simulink model "AUAV_V3_TestSensors"  (Simulink 8.5)
settings: Solver=FixedStepDiscrete  StartTime=0.0  StopTime=10.0  FixedStep=T  RelTol=1e-3
PreLoadFcn:
  | %T = 0.0025;
  | MavlinkBus;
  | mcuInit;
  | % Baro Altitude Computation
  | % =========================
  | basePressure = 98192.64;
  | baseTemp = 288.215;
  | lapseRate = -0.00198122;
  | baseHeight = 0;
undefined symbols (not defined in the file): A0, A14, A15, A2, A3, A4, A5, A6, accBiasRateLimit, apSampleTime, B0, bankCommandLimit, barAdjust, baroCutoff, baroCutTemp, baroOffset, baroScale, barTGain1, barTGain2, barTMean1, barTMean2, bda, bde, bdr, bdt, bICda, bICde, bICdr, bICdt, cubeAccelGain16405, cubeGyroGain16405, cubeMagGain16405, D0, D11, D7, D8, daLimit, data, daTrimMax, daTrimMin, deLimit, derivativesConstant, deTrimMax, deTrimMin, drLimit, drTrimMax, drTrimMin, dtLimit, dtTrimMax, dtTrimMin, F2, F3, G0, G13, G15, gaind, GS_location, gyroBiasRateLimit, IC1max, IPStar ... (+71)
libraries: MCHP_Blockset x152, simulink x84, SLUGS_Library x31, aerolibconvert2 x6, aerolibutil x4, aerolibtransform2 x3, dspmtrx3 x2, aerolibobsolete x2
(part 19 of 20)

== system AUAV_V3_TestSensors/Inner Loop/ Navigation/Navigation Encaps [updated 4.28.16]/Navigation/Normal WP  Navigation/Get Frenet/get WP Coord from Index2 ==
  WP Idx : Inport
  GS LLA : Inport  Port=2
  GS R_in : Inport  Port=3
  Demux1 : Demux  Outputs=3
  Environment Controller1 : simulink/Signal Routing/Environment Controller
  Geod2LTP2 : SLUGS_Library/Navigation/Geod2LTP
  Get WP Coord navsupport.c [updated 5.1.16] : MCHP_Blockset/User Functions/C Function Call  ParseFilesChkbx=off  ListFunctions1=Custom Function  Function1=void getWP(unsigned char idx, float* WPpos)  AddHeaderDeclaration=on  Function1Type=when block is updated (default)  Fct1BlockIn=idx  FctReturnBlockOut=on  Fct1BlockOut=WPpos[3]  DataCollected=0  ORDERING=None  SampleTime=-1  MCHP_MASTERLINK=|  PinDigitalInput=[]  PinDigitalOutput=[]  PinAnalogInput=[]
      | AUAV_V3_TestSensors/Microchip Master
      | AUAV V3 Board
      | Busy Flag on D2 (RA6)
  Get WP from idx SIM : Subsystem
  WP Coord : Outport
  wires:
  Geod2LTP2/1 -> Environment Controller1/2
  Get WP Coord navsupport.c [updated 5.1.16]/1 -> Demux1/1
  Demux1/3 -> Geod2LTP2/5
  Demux1/2 -> Geod2LTP2/4
  Demux1/1 -> Geod2LTP2/3
  Get WP from idx SIM/1(Out1) -> Environment Controller1/1
  Environment Controller1/1 -> WP Coord/1
  GS R_in/1 -> Get WP from idx SIM/2(GS ECEF), Geod2LTP2/2
  GS LLA/1 -> Get WP from idx SIM/1(GS LLA), Geod2LTP2/1
  WP Idx/1 -> Get WP from idx SIM/3(idx), Get WP Coord navsupport.c [updated 5.1.16]/1

== system AUAV_V3_TestSensors/Inner Loop/ Navigation/Navigation Encaps [updated 4.28.16]/Navigation/Normal WP  Navigation/On WP Enable/Subsystem ==
  GS LLA : Inport
  GS R_in : Inport  Port=2
  Compute Frenet : Subsystem  AncestorBlock=SLUGS_Library/Navigation/Compute Frenet
  Constant : Constant  OutDataTypeStr=uint8  SampleTime=0.01
  Constant1 : Constant  Value=2  OutDataTypeStr=uint8  SampleTime=0.01
  GS LLA_1 : InportShadow
  GS R_in_1 : InportShadow  Port=2
  Terminator : Terminator
  get WP Coord from Index : Subsystem  AncestorBlock=SLUGS_Library/Navigation/get WP Coord from Index
  get WP Coord from Index1 : Subsystem  AncestorBlock=SLUGS_Library/Navigation/get WP Coord from Index
  WP0 : Outport
  T1 : Outport  Port=2
  wires:
  Constant/1 -> get WP Coord from Index/1(WP Idx)
  Compute Frenet/2(N) -> Terminator/1
  Compute Frenet/1(T) -> T1/1
  GS LLA/1 -> get WP Coord from Index/2(GS LLA)
  GS R_in/1 -> get WP Coord from Index/3(GS R_in)
  get WP Coord from Index/1(WP Coord) -> WP0/1, Compute Frenet/1(Pos 1)
  get WP Coord from Index1/1(WP Coord) -> Compute Frenet/2(Pos 2)
  Constant1/1 -> get WP Coord from Index1/1(WP Idx)
  GS LLA_1/1 -> get WP Coord from Index1/2(GS LLA)
  GS R_in_1/1 -> get WP Coord from Index1/3(GS R_in)

== system AUAV_V3_TestSensors/Inner Loop/ Navigation/Navigation Encaps [updated 4.28.16]/Navigation/Normal WP  Navigation/Vector Norm/dsPIC_SQRT ==
  x : Inport
  Environment Controller : simulink/Signal Routing/Environment Controller
  Math Function1 : Math  Operator=sqrt  SaturateOnIntegerOverflow=on
  mySqrt() apUtils.c [updated 5.1.16] : MCHP_Blockset/User Functions/C Function Call  ParseFilesChkbx=off  ListFunctions1=Custom Function  Function1=float mySqrt(float x)  AddHeaderDeclaration=on  Function1Type=when block is updated (default)  Fct1BlockIn=x  FctReturnBlockOut=on  DataCollected=0  ORDERING=None  SampleTime=-1  MCHP_MASTERLINK=|  PinDigitalInput=[]  PinDigitalOutput=[]  PinAnalogInput=[]
      | AUAV_V3_TestSensors/Microchip Master
      | AUAV V3 Board
      | Busy Flag on D2 (RA6)
  negprotect : MATLAB Function  TreatAsAtomicUnit=on
  sqrt(x) : Outport
  wires:
  x/1 -> negprotect/1(val)
  negprotect/1(zpVal) -> Math Function1/1, mySqrt() apUtils.c [updated 5.1.16]/1
  Environment Controller/1 -> sqrt(x)/1
  Math Function1/1 -> Environment Controller/1
  mySqrt() apUtils.c [updated 5.1.16]/1 -> Environment Controller/2

== system AUAV_V3_TestSensors/Inner Loop/ Navigation/Navigation Encaps [updated 4.28.16]/Navigation/RTB/Follow Mobile Navigation/Vector Norm/dsPIC_SQRT ==
  x : Inport
  Environment Controller : simulink/Signal Routing/Environment Controller
  Math Function1 : Math  Operator=sqrt  SaturateOnIntegerOverflow=on
  mySqrt() apUtils.c [updated 5.1.16] : MCHP_Blockset/User Functions/C Function Call  ParseFilesChkbx=off  ListFunctions1=Custom Function  Function1=float mySqrt(float x)  AddHeaderDeclaration=on  Function1Type=when block is updated (default)  Fct1BlockIn=x  FctReturnBlockOut=on  DataCollected=0  ORDERING=None  SampleTime=-1  MCHP_MASTERLINK=|  PinDigitalInput=[]  PinDigitalOutput=[]  PinAnalogInput=[]
      | AUAV_V3_TestSensors/Microchip Master
      | AUAV V3 Board
      | Busy Flag on D2 (RA6)
  negprotect : MATLAB Function  TreatAsAtomicUnit=on
  sqrt(x) : Outport
  wires:
  x/1 -> negprotect/1(val)
  negprotect/1(zpVal) -> Math Function1/1, mySqrt() apUtils.c [updated 5.1.16]/1
  Environment Controller/1 -> sqrt(x)/1
  Math Function1/1 -> Environment Controller/1
  mySqrt() apUtils.c [updated 5.1.16]/1 -> Environment Controller/2

== system AUAV_V3_TestSensors/Inner Loop/ Navigation/Navigation Encaps [updated 4.28.16]/Navigation/Recent Enable/Grab Upon Enable/Compute GS Location ==
  GS Location : Inport
  Demux : Demux  Outputs=3
  Geod2ECEF1 : Subsystem  mask{Re=6378137, Rp=6356752.3142}
      mask prompts: Re "Enter equatorial radius, m"; Rp "Enter polar radius,m"
  Mux1 : Mux  Inputs=2
  Mux2 : Mux  Inputs=3
  "Lon, Lat" : Outport
  R_in : Outport  Port=2
  wires:
  Mux2/1 -> R_in/1  "R_in"
  Mux1/1 -> "Lon, Lat"/1
  GS Location/1 -> Demux/1
  Demux/3 -> Mux1/1, Geod2ECEF1/3(lon,deg)
  Demux/2 -> Mux1/2, Geod2ECEF1/2("lat, deg")
  Demux/1 -> Geod2ECEF1/1("height, m")
  Geod2ECEF1/2("Ye, m ") -> Mux2/2
  Geod2ECEF1/1("Xe, m ") -> Mux2/1
  Geod2ECEF1/3("Ze, m ") -> Mux2/3

== system AUAV_V3_TestSensors/Inner Loop/ Navigation/Navigation Encaps [updated 4.28.16]/Navigation/Recent Enable/Subsystem/Detect Rising Edge ==
  In1 : Inport
  Delay : Delay  DelayLength=1
  Logical Operator : Logic  AllPortsSameDT=off  OutDataTypeStr=boolean
  Relational Operator : RelationalOperator  Operator=~=  OutDataTypeStr=boolean
  Out1 : Outport
  wires:
  Delay/1 -> Relational Operator/1
  Relational Operator/1 -> Logical Operator/1
  In1/1 -> Delay/1, Relational Operator/2, Logical Operator/2
  Logical Operator/1 -> Out1/1

== system AUAV_V3_TestSensors/Position_and_Attitude_Filter/Position Filter/BlendPosVel/CompFiltRate/1D Filter1/Filter2 ==
  In1 : Inport
  Discrete Zero-Pole : DiscreteZeroPole  Zeros=zerosd  Poles=polesd  Gain=gaind  SampleTime=SampleTime
  Out1 : Outport
  wires:
  Discrete Zero-Pole/1 -> Out1/1
  In1/1 -> Discrete Zero-Pole/1

== system AUAV_V3_TestSensors/Position_and_Attitude_Filter/Position Filter/BlendPosVel/CompFiltRate1/1D Filter1/Filter2 ==
  In1 : Inport
  Discrete Zero-Pole : DiscreteZeroPole  Zeros=zerosd  Poles=polesd  Gain=gaind  SampleTime=SampleTime
  Out1 : Outport
  wires:
  Discrete Zero-Pole/1 -> Out1/1
  In1/1 -> Discrete Zero-Pole/1

== system AUAV_V3_TestSensors/Position_and_Attitude_Filter/Position Filter/BlendPosVel/CompRateOnly/1D Filter1/Filter2 ==
  In1 : Inport
  Discrete Zero-Pole : DiscreteZeroPole  Zeros=zerosd  Poles=polesd  Gain=gaind  SampleTime=SampleTime
  Out1 : Outport
  wires:
  Discrete Zero-Pole/1 -> Out1/1
  In1/1 -> Discrete Zero-Pole/1

== system AUAV_V3_TestSensors/Sensor_Data_Adapter/Sensor Suite/Low Pass Filtering,Temperature Compensation and Calibration/Baro Altimeter/Initial Baro Bias/Low Pass8 ==
  In1 : Inport
  Discrete Zero-Pole : DiscreteZeroPole  Zeros=zerosd  Poles=polesd  Gain=gaind  SampleTime=SampleTime
  Out1 : Outport
  wires:
  In1/1 -> Discrete Zero-Pole/1
  Discrete Zero-Pole/1 -> Out1/1

== system AUAV_V3_TestSensors/Inner Loop/ Navigation/Navigation Encaps [updated 4.28.16]/Navigation/Circle Navigation/Intersection. Circular Navigation/Compute Angle Between Vectors1/Vector Norm ==
  Vector : Inport
  dsPIC Dot Product : SLUGS_Library/dsPIC Dot Product
  dsPIC_SQRT : Subsystem  AncestorBlock=SLUGS_Library/dsPIC_SQRT
  Norm : Outport
  wires:
  dsPIC_SQRT/1(sqrt(x)) -> Norm/1
  Vector/1 -> dsPIC Dot Product/2, dsPIC Dot Product/1
  dsPIC Dot Product/1 -> dsPIC_SQRT/1(x)

== system AUAV_V3_TestSensors/Inner Loop/ Navigation/Navigation Encaps [updated 4.28.16]/Navigation/Circle Navigation/Intersection. Circular Navigation/Compute Angle Between Vectors1/dsPIC_acos ==
  x : Inport
  Environment Controller : simulink/Signal Routing/Environment Controller
  Trigonometric Function : Trigonometry  Operator=acos
  myAcos() apUtils.c [updated 5.1.16] : MCHP_Blockset/User Functions/C Function Call  ParseFilesChkbx=off  ListFunctions1=Custom Function  Function1=float myAcos(float x)  AddHeaderDeclaration=off  Function1Type=when block is updated (default)  Fct1BlockIn=x  FctReturnBlockOut=on  DataCollected=0  ORDERING=None  SampleTime=-1  MCHP_MASTERLINK=|  PinDigitalInput=[]  PinDigitalOutput=[]  PinAnalogInput=[]
      | AUAV_V3_TestSensors/Microchip Master
      | AUAV V3 Board
      | Busy Flag on D2 (RA6)
  acos(x) : Outport
  wires:
  Environment Controller/1 -> acos(x)/1
  myAcos() apUtils.c [updated 5.1.16]/1 -> Environment Controller/2
  Trigonometric Function/1 -> Environment Controller/1
  x/1 -> Trigonometric Function/1, myAcos() apUtils.c [updated 5.1.16]/1

== system AUAV_V3_TestSensors/Inner Loop/ Navigation/Navigation Encaps [updated 4.28.16]/Navigation/Circle Navigation/Intersection. Circular Navigation/Compute Angle Between Vectors2/Vector Norm ==
  Vector : Inport
  dsPIC Dot Product : SLUGS_Library/dsPIC Dot Product
  dsPIC_SQRT : Subsystem  AncestorBlock=SLUGS_Library/dsPIC_SQRT
  Norm : Outport
  wires:
  dsPIC_SQRT/1(sqrt(x)) -> Norm/1
  Vector/1 -> dsPIC Dot Product/2, dsPIC Dot Product/1
  dsPIC Dot Product/1 -> dsPIC_SQRT/1(x)

== system AUAV_V3_TestSensors/Inner Loop/ Navigation/Navigation Encaps [updated 4.28.16]/Navigation/Circle Navigation/Intersection. Circular Navigation/Compute Angle Between Vectors2/dsPIC_acos ==
  x : Inport
  Environment Controller : simulink/Signal Routing/Environment Controller
  Trigonometric Function : Trigonometry  Operator=acos
  myACos() apUtils.c [updated 5.1.16] : MCHP_Blockset/User Functions/C Function Call  ParseFilesChkbx=off  ListFunctions1=Custom Function  Function1=float myAcos(float x)  AddHeaderDeclaration=off  Function1Type=when block is updated (default)  Fct1BlockIn=x  FctReturnBlockOut=on  DataCollected=0  ORDERING=None  SampleTime=-1  MCHP_MASTERLINK=|  PinDigitalInput=[]  PinDigitalOutput=[]  PinAnalogInput=[]
      | AUAV_V3_TestSensors/Microchip Master
      | AUAV V3 Board
      | Busy Flag on D2 (RA6)
  acos(x) : Outport
  wires:
  Environment Controller/1 -> acos(x)/1
  myACos() apUtils.c [updated 5.1.16]/1 -> Environment Controller/2
  Trigonometric Function/1 -> Environment Controller/1
  x/1 -> Trigonometric Function/1, myACos() apUtils.c [updated 5.1.16]/1

== system AUAV_V3_TestSensors/Inner Loop/ Navigation/Navigation Encaps [updated 4.28.16]/Navigation/L2+/Get Sin, Cos eta/Get  Groundspeed/Vector Norm ==
  Vector : Inport
  dsPIC Dot Product : SLUGS_Library/dsPIC Dot Product
  dsPIC_SQRT : Subsystem  AncestorBlock=SLUGS_Library/dsPIC_SQRT
  Norm : Outport
  wires:
  dsPIC_SQRT/1(sqrt(x)) -> Norm/1
  Vector/1 -> dsPIC Dot Product/2, dsPIC Dot Product/1
  dsPIC Dot Product/1 -> dsPIC_SQRT/1(x)

== system AUAV_V3_TestSensors/Inner Loop/ Navigation/Navigation Encaps [updated 4.28.16]/Navigation/Normal WP  Navigation/Compute WP Switching Trigger/Compute  Projection/Protect NaNs ==
  In1 : Inport
  Integer Delay3 : Delay  DelayLength=1  InputProcessing=Inherited  SampleTime=T
  Relational Operator2 : RelationalOperator  Operator===  OutDataTypeStr=uint(8)
  Switch3 : Switch  Criteria=u2 > Threshold  Threshold=0.3  SampleTime=.01
  Out1 : Outport
  wires:
  Relational Operator2/1 -> Switch3/2
  In1/1 -> Switch3/1, Relational Operator2/1, Relational Operator2/2
  Switch3/1 -> Integer Delay3/1, Out1/1
  Integer Delay3/1 -> Switch3/3

== system AUAV_V3_TestSensors/Inner Loop/ Navigation/Navigation Encaps [updated 4.28.16]/Navigation/Normal WP  Navigation/Get Frenet/Compute Frenet/Normalize Vector ==
  Vector : Inport
  Divide : Product  Inputs=*/
  Vector Norm : Subsystem  AncestorBlock=SLUGS_Library/Vector Norm
  Zero Bound : Saturate  UpperLimit=inf  LowerLimit=0.001
  Normalized : Outport
  wires:
  Vector/1 -> Vector Norm/1(Vector), Divide/1
  Vector Norm/1(Norm) -> Zero Bound/1
  Zero Bound/1 -> Divide/2
  Divide/1 -> Normalized/1

== system AUAV_V3_TestSensors/Inner Loop/ Navigation/Navigation Encaps [updated 4.28.16]/Navigation/Normal WP  Navigation/Get Frenet/Compute Frenet/Normalize Vector  ==
  Vector : Inport
  Divide : Product  Inputs=*/
  Vector Norm : Subsystem  AncestorBlock=SLUGS_Library/Vector Norm
  Zero Bound : Saturate  UpperLimit=inf  LowerLimit=0.001
  Normalized : Outport
  wires:
  Vector/1 -> Vector Norm/1(Vector), Divide/1
  Vector Norm/1(Norm) -> Zero Bound/1
  Zero Bound/1 -> Divide/2
  Divide/1 -> Normalized/1

== system AUAV_V3_TestSensors/Inner Loop/ Navigation/Navigation Encaps [updated 4.28.16]/Navigation/Normal WP  Navigation/Get Frenet/get WP Coord from Index1/Get WP from idx SIM ==
  GS LLA : Inport
  GS ECEF : Inport  Port=2
  idx : Inport  Port=3
  Constant : Constant  Value=latlong_WP  OutDataTypeStr=uint8  SampleTime=0.01
  Constant1 : Constant  Value=Ypoints  OutDataTypeStr=double  SampleTime=0.01
  Constant2 : Constant  Value=Xpoints  OutDataTypeStr=double  SampleTime=0.01
  Constant3 : Constant  Value=Zpoints  OutDataTypeStr=double  SampleTime=0.01
  Data Type Conversion : DataTypeConversion  OutDataTypeStr=double
  Data Type Conversion1 : DataTypeConversion  OutDataTypeStr=single
  Demux : Demux  Outputs=3
  Geod2LTP1 : SLUGS_Library/Navigation/Geod2LTP
  Mux : Mux  Inputs=3
  Switch : Switch  Criteria=u2 > Threshold  Threshold=0.3  ZeroCross=off
  Zero out Z1 : MATLAB Function  TreatAsAtomicUnit=on
  Zero out Z2 : MATLAB Function  TreatAsAtomicUnit=on
  Zero out Z3 : MATLAB Function  TreatAsAtomicUnit=on
  Out1 : Outport
  wires:
  Constant2/1 -> Zero out Z2/2(vect)
  Constant3/1 -> Zero out Z3/2(vect)
  Constant1/1 -> Zero out Z1/2(vect)
  Switch/1 -> Out1/1
  idx/1 -> Data Type Conversion/1
  GS ECEF/1 -> Geod2LTP1/2
  GS LLA/1 -> Geod2LTP1/1
  Data Type Conversion1/1 -> Demux/1, Switch/3
  Geod2LTP1/1 -> Switch/1
  Demux/3 -> Geod2LTP1/5
  Demux/2 -> Geod2LTP1/4
  Demux/1 -> Geod2LTP1/3
  Constant/1 -> Switch/2
  Mux/1 -> Data Type Conversion1/1
  Zero out Z3/1(y) -> Mux/3
  Zero out Z1/1(y) -> Mux/2
  Zero out Z2/1(y) -> Mux/1
  Data Type Conversion/1 -> Zero out Z3/1(idx), Zero out Z1/1(idx), Zero out Z2/1(idx)

== system AUAV_V3_TestSensors/Inner Loop/ Navigation/Navigation Encaps [updated 4.28.16]/Navigation/Normal WP  Navigation/Get Frenet/get WP Coord from Index2/Get WP from idx SIM ==
  GS LLA : Inport
  GS ECEF : Inport  Port=2
  idx : Inport  Port=3
  Constant : Constant  Value=latlong_WP  OutDataTypeStr=uint8  SampleTime=0.01
  Constant1 : Constant  Value=Ypoints  OutDataTypeStr=double  SampleTime=0.01
  Constant2 : Constant  Value=Xpoints  OutDataTypeStr=double  SampleTime=0.01
  Constant3 : Constant  Value=Zpoints  OutDataTypeStr=double  SampleTime=0.01
  Data Type Conversion : DataTypeConversion  OutDataTypeStr=double
  Data Type Conversion1 : DataTypeConversion  OutDataTypeStr=single
  Demux : Demux  Outputs=3
  Geod2LTP1 : SLUGS_Library/Navigation/Geod2LTP
  Mux : Mux  Inputs=3
  Switch : Switch  Criteria=u2 > Threshold  Threshold=0.3  ZeroCross=off
  Zero out Z1 : MATLAB Function  TreatAsAtomicUnit=on
  Zero out Z2 : MATLAB Function  TreatAsAtomicUnit=on
  Zero out Z3 : MATLAB Function  TreatAsAtomicUnit=on
  Out1 : Outport
  wires:
  Constant2/1 -> Zero out Z2/2(vect)
  Constant3/1 -> Zero out Z3/2(vect)
  Constant1/1 -> Zero out Z1/2(vect)
  Switch/1 -> Out1/1
  idx/1 -> Data Type Conversion/1
  GS ECEF/1 -> Geod2LTP1/2
  GS LLA/1 -> Geod2LTP1/1
  Data Type Conversion1/1 -> Demux/1, Switch/3
  Geod2LTP1/1 -> Switch/1
  Demux/3 -> Geod2LTP1/5
  Demux/2 -> Geod2LTP1/4
  Demux/1 -> Geod2LTP1/3
  Constant/1 -> Switch/2
  Mux/1 -> Data Type Conversion1/1
  Zero out Z3/1(y) -> Mux/3
  Zero out Z1/1(y) -> Mux/2
  Zero out Z2/1(y) -> Mux/1
  Data Type Conversion/1 -> Zero out Z3/1(idx), Zero out Z1/1(idx), Zero out Z2/1(idx)

== system AUAV_V3_TestSensors/Inner Loop/ Navigation/Navigation Encaps [updated 4.28.16]/Navigation/Normal WP  Navigation/On WP Enable/Subsystem/Compute Frenet ==
  Pos 1 : Inport
  Pos 2 : Inport  Port=2
  Add : Sum  Inputs=-+
  Normalize Vector : Subsystem  AncestorBlock=SLUGS_Library/Navigation/Normalize Vector
  "Normalize Vector " : Subsystem  AncestorBlock=SLUGS_Library/Navigation/Normalize Vector
  Select N  Terms : MATLAB Function  TreatAsAtomicUnit=on
  T : Outport
  N : Outport  Port=2
  wires:
  "Normalize Vector "/1(Normalized) -> N/1
  Select N  Terms/1(N) -> "Normalize Vector "/1(Vector)
  Normalize Vector/1(Normalized) -> Select N  Terms/1(T), T/1
  Add/1 -> Normalize Vector/1(Vector)
  Pos 2/1 -> Add/2
  Pos 1/1 -> Add/1

== system AUAV_V3_TestSensors/Inner Loop/ Navigation/Navigation Encaps [updated 4.28.16]/Navigation/Normal WP  Navigation/On WP Enable/Subsystem/get WP Coord from Index ==
  WP Idx : Inport
  GS LLA : Inport  Port=2
  GS R_in : Inport  Port=3
  Demux1 : Demux  Outputs=3
  Environment Controller1 : simulink/Signal Routing/Environment Controller
  Geod2LTP2 : SLUGS_Library/Navigation/Geod2LTP
  Get WP Coord navsupport.c [updated 5.1.16] : MCHP_Blockset/User Functions/C Function Call  ParseFilesChkbx=off  ListFunctions1=Custom Function  Function1=void getWP(unsigned char idx, float* WPpos)  AddHeaderDeclaration=on  Function1Type=when block is updated (default)  Fct1BlockIn=idx  FctReturnBlockOut=on  Fct1BlockOut=WPpos[3]  DataCollected=0  ORDERING=None  SampleTime=-1  MCHP_MASTERLINK=|  PinDigitalInput=[]  PinDigitalOutput=[]  PinAnalogInput=[]
      | AUAV_V3_TestSensors/Microchip Master
      | AUAV V3 Board
      | Busy Flag on D2 (RA6)
  Get WP from idx SIM : Subsystem
  WP Coord : Outport
  wires:
  Geod2LTP2/1 -> Environment Controller1/2
  Get WP Coord navsupport.c [updated 5.1.16]/1 -> Demux1/1
  Demux1/3 -> Geod2LTP2/5
  Demux1/2 -> Geod2LTP2/4
  Demux1/1 -> Geod2LTP2/3
  Get WP from idx SIM/1(Out1) -> Environment Controller1/1
  Environment Controller1/1 -> WP Coord/1
  GS R_in/1 -> Get WP from idx SIM/2(GS ECEF), Geod2LTP2/2
  GS LLA/1 -> Get WP from idx SIM/1(GS LLA), Geod2LTP2/1
  WP Idx/1 -> Get WP from idx SIM/3(idx), Get WP Coord navsupport.c [updated 5.1.16]/1

== system AUAV_V3_TestSensors/Inner Loop/ Navigation/Navigation Encaps [updated 4.28.16]/Navigation/Normal WP  Navigation/On WP Enable/Subsystem/get WP Coord from Index1 ==
  WP Idx : Inport
  GS LLA : Inport  Port=2
  GS R_in : Inport  Port=3
  Demux1 : Demux  Outputs=3
  Environment Controller1 : simulink/Signal Routing/Environment Controller
  Geod2LTP2 : SLUGS_Library/Navigation/Geod2LTP
  Get WP Coord navsupport.c [updated 5.1.16] : MCHP_Blockset/User Functions/C Function Call  ParseFilesChkbx=off  ListFunctions1=Custom Function  Function1=void getWP(unsigned char idx, float* WPpos)  AddHeaderDeclaration=on  Function1Type=when block is updated (default)  Fct1BlockIn=idx  FctReturnBlockOut=on  Fct1BlockOut=WPpos[3]  DataCollected=0  ORDERING=None  SampleTime=-1  MCHP_MASTERLINK=|  PinDigitalInput=[]  PinDigitalOutput=[]  PinAnalogInput=[]
      | AUAV_V3_TestSensors/Microchip Master
      | AUAV V3 Board
      | Busy Flag on D2 (RA6)
  Get WP from idx SIM : Subsystem
  WP Coord : Outport
  wires:
  Geod2LTP2/1 -> Environment Controller1/2
  Get WP Coord navsupport.c [updated 5.1.16]/1 -> Demux1/1
  Demux1/3 -> Geod2LTP2/5
  Demux1/2 -> Geod2LTP2/4
  Demux1/1 -> Geod2LTP2/3
  Get WP from idx SIM/1(Out1) -> Environment Controller1/1
  Environment Controller1/1 -> WP Coord/1
  GS R_in/1 -> Get WP from idx SIM/2(GS ECEF), Geod2LTP2/2
  GS LLA/1 -> Get WP from idx SIM/1(GS LLA), Geod2LTP2/1
  WP Idx/1 -> Get WP from idx SIM/3(idx), Get WP Coord navsupport.c [updated 5.1.16]/1

== system AUAV_V3_TestSensors/Inner Loop/ Navigation/Navigation Encaps [updated 4.28.16]/Navigation/Recent Enable/Grab Upon Enable/Compute GS Location/Geod2ECEF1 ==
  "height, m" : Inport
  "lat, deg" : Inport  Port=2
  lon,deg : Inport  Port=3
  (Rh+h)cos(phi)*cos(lamb)=Xe : Product  Inputs=3  OutDataTypeStr=single  SaturateOnIntegerOverflow=on  InputSameDT=on
  (Rh+h)cos(phi)*sin(lamb)=Ye : Product  Inputs=3  OutDataTypeStr=single  SaturateOnIntegerOverflow=on  InputSameDT=on
  Deg2R : Gain  Gain=pi/180  OutDataTypeStr=float('single')  SaturateOnIntegerOverflow=on  ParamDataTypeStr=Inherit: Same as input
  Deg2R1 : Gain  Gain=pi/180  OutDataTypeStr=float('single')  SaturateOnIntegerOverflow=on  ParamDataTypeStr=Inherit: Same as input
  Product1 : Product  SaturateOnIntegerOverflow=on  InputSameDT=on  OutDataTypeStr=Inherit: Same as first input
  Re=equatorial radius : Constant  Value=Re  OutDataTypeStr=single
  Rh : Product  Inputs=*/  OutDataTypeStr=single  SaturateOnIntegerOverflow=on  InputSameDT=on
  Rh(1-e^2) : Product  OutDataTypeStr=single  SaturateOnIntegerOverflow=on  InputSameDT=on
  Sum1 : Sum  Inputs=+-|  SaturateOnIntegerOverflow=on  InputSameDT=on  OutDataTypeStr=Inherit: Same as first input
  Sum2 : Sum  SaturateOnIntegerOverflow=on  InputSameDT=on  OutDataTypeStr=Inherit: Same as first input
      settings: AttributesFormatString=Rh+h
  Sum3 : Sum  Inputs=|+-  SaturateOnIntegerOverflow=on  InputSameDT=on  OutDataTypeStr=Inherit: Same as first input
  Sum4 : Sum  OutDataTypeStr=single  SaturateOnIntegerOverflow=on  InputSameDT=on
      settings: AttributesFormatString=(1-e^2)Rh+h
  Ze : Product  OutDataTypeStr=single  SaturateOnIntegerOverflow=on  InputSameDT=on
  const : Constant  OutDataTypeStr=single
  const1 : Constant  OutDataTypeStr=single
  cos(lamb) : Trigonometry  Operator=cos
  cos(phi) : Trigonometry  Operator=cos
  eccentricity^2 : Subsystem
  f : Fcn  Expr=sqrt(u(1))
  sin(lamb) : Trigonometry
  sin(phi) : Trigonometry
  sin(phi)^2 : Product  SaturateOnIntegerOverflow=on  InputSameDT=on  OutDataTypeStr=Inherit: Same as first input
  "Xe, m " : Outport
  "Ye, m " : Outport  Port=2
  "Ze, m " : Outport  Port=3
  wires:
  "lat, deg"/1 -> Deg2R/1
  sin(phi)/1 -> sin(phi)^2/1, sin(phi)^2/2, Ze/1
  f/1 -> Rh/2
  Re=equatorial radius/1 -> Rh/1
  Rh/1 -> Sum2/2, Rh(1-e^2)/2
  Product1/1 -> Sum1/2
  Sum1/1 -> f/1
  const/1 -> Sum1/1
  "height, m"/1 -> Sum4/2, Sum2/1
  eccentricity^2/1(e^2) -> Product1/1, Sum3/2
  sin(phi)^2/1 -> Product1/2
  const1/1 -> Sum3/1
  Sum3/1 -> Rh(1-e^2)/1  "1-e^2"
  Rh(1-e^2)/1 -> Sum4/1
  Sum4/1 -> Ze/2
  lon,deg/1 -> Deg2R1/1
  cos(phi)/1 -> (Rh+h)cos(phi)*cos(lamb)=Xe/2, (Rh+h)cos(phi)*sin(lamb)=Ye/2
  cos(lamb)/1 -> (Rh+h)cos(phi)*cos(lamb)=Xe/3
  sin(lamb)/1 -> (Rh+h)cos(phi)*sin(lamb)=Ye/3
  Ze/1 -> "Ze, m "/1
  Deg2R/1 -> cos(phi)/1, sin(phi)/1
  Deg2R1/1 -> cos(lamb)/1, sin(lamb)/1
  Sum2/1 -> (Rh+h)cos(phi)*sin(lamb)=Ye/1, (Rh+h)cos(phi)*cos(lamb)=Xe/1
  (Rh+h)cos(phi)*cos(lamb)=Xe/1 -> "Xe, m "/1
  (Rh+h)cos(phi)*sin(lamb)=Ye/1 -> "Ye, m "/1

== system AUAV_V3_TestSensors/Inner Loop/ Navigation/Navigation Encaps [updated 4.28.16]/Navigation/Circle Navigation/Intersection. Circular Navigation/Compute Angle Between Vectors1/Vector Norm/dsPIC_SQRT ==
  x : Inport
  Environment Controller : simulink/Signal Routing/Environment Controller
  Math Function1 : Math  Operator=sqrt  SaturateOnIntegerOverflow=on
  mySqrt() apUtils.c [updated 5.1.16] : MCHP_Blockset/User Functions/C Function Call  ParseFilesChkbx=off  ListFunctions1=Custom Function  Function1=float mySqrt(float x)  AddHeaderDeclaration=off  Function1Type=when block is updated (default)  Fct1BlockIn=x  FctReturnBlockOut=on  DataCollected=0  ORDERING=None  SampleTime=-1  MCHP_MASTERLINK=|  PinDigitalInput=[]  PinDigitalOutput=[]  PinAnalogInput=[]
      | AUAV_V3_TestSensors/Microchip Master
      | AUAV V3 Board
      | Busy Flag on D2 (RA6)
  negprotect : MATLAB Function  TreatAsAtomicUnit=on
  sqrt(x) : Outport
  wires:
  x/1 -> negprotect/1(val)
  negprotect/1(zpVal) -> Math Function1/1, mySqrt() apUtils.c [updated 5.1.16]/1
  Environment Controller/1 -> sqrt(x)/1
  Math Function1/1 -> Environment Controller/1
  mySqrt() apUtils.c [updated 5.1.16]/1 -> Environment Controller/2

== system AUAV_V3_TestSensors/Inner Loop/ Navigation/Navigation Encaps [updated 4.28.16]/Navigation/Circle Navigation/Intersection. Circular Navigation/Compute Angle Between Vectors2/Vector Norm/dsPIC_SQRT ==
  x : Inport
  Environment Controller : simulink/Signal Routing/Environment Controller
  Math Function1 : Math  Operator=sqrt  SaturateOnIntegerOverflow=on
  mySqrt() apUtils.c [updated 5.1.16] : MCHP_Blockset/User Functions/C Function Call  ParseFilesChkbx=off  ListFunctions1=Custom Function  Function1=float mySqrt(float x)  AddHeaderDeclaration=off  Function1Type=when block is updated (default)  Fct1BlockIn=x  FctReturnBlockOut=on  DataCollected=0  ORDERING=None  SampleTime=-1  MCHP_MASTERLINK=|  PinDigitalInput=[]  PinDigitalOutput=[]  PinAnalogInput=[]
      | AUAV_V3_TestSensors/Microchip Master
      | AUAV V3 Board
      | Busy Flag on D2 (RA6)
  negprotect : MATLAB Function  TreatAsAtomicUnit=on
  sqrt(x) : Outport
  wires:
  x/1 -> negprotect/1(val)
  negprotect/1(zpVal) -> Math Function1/1, mySqrt() apUtils.c [updated 5.1.16]/1
  Environment Controller/1 -> sqrt(x)/1
  Math Function1/1 -> Environment Controller/1
  mySqrt() apUtils.c [updated 5.1.16]/1 -> Environment Controller/2

== system AUAV_V3_TestSensors/Inner Loop/ Navigation/Navigation Encaps [updated 4.28.16]/Navigation/L2+/Get Sin, Cos eta/Get  Groundspeed/Vector Norm/dsPIC_SQRT ==
  x : Inport
  Environment Controller : simulink/Signal Routing/Environment Controller
  Math Function1 : Math  Operator=sqrt  SaturateOnIntegerOverflow=on
  mySqrt() apUtils.c [updated 5.1.16] : MCHP_Blockset/User Functions/C Function Call  ParseFilesChkbx=off  ListFunctions1=Custom Function  Function1=float mySqrt(float x)  AddHeaderDeclaration=on  Function1Type=when block is updated (default)  Fct1BlockIn=x  FctReturnBlockOut=on  DataCollected=0  ORDERING=None  SampleTime=-1  MCHP_MASTERLINK=|  PinDigitalInput=[]  PinDigitalOutput=[]  PinAnalogInput=[]
      | AUAV_V3_TestSensors/Microchip Master
      | AUAV V3 Board
      | Busy Flag on D2 (RA6)
  negprotect : MATLAB Function  TreatAsAtomicUnit=on
  sqrt(x) : Outport
  wires:
  x/1 -> negprotect/1(val)
  negprotect/1(zpVal) -> Math Function1/1, mySqrt() apUtils.c [updated 5.1.16]/1
  Environment Controller/1 -> sqrt(x)/1
  Math Function1/1 -> Environment Controller/1
  mySqrt() apUtils.c [updated 5.1.16]/1 -> Environment Controller/2

== system AUAV_V3_TestSensors/Inner Loop/ Navigation/Navigation Encaps [updated 4.28.16]/Navigation/Normal WP  Navigation/Get Frenet/Compute Frenet/Normalize Vector/Vector Norm ==
  Vector : Inport
  dsPIC Dot Product : SLUGS_Library/dsPIC Dot Product
  dsPIC_SQRT : Subsystem  AncestorBlock=SLUGS_Library/dsPIC_SQRT
  Norm : Outport
  wires:
  dsPIC_SQRT/1(sqrt(x)) -> Norm/1
  Vector/1 -> dsPIC Dot Product/2, dsPIC Dot Product/1
  dsPIC Dot Product/1 -> dsPIC_SQRT/1(x)

== system AUAV_V3_TestSensors/Inner Loop/ Navigation/Navigation Encaps [updated 4.28.16]/Navigation/Normal WP  Navigation/Get Frenet/Compute Frenet/Normalize Vector /Vector Norm ==
  Vector : Inport
  dsPIC Dot Product : SLUGS_Library/dsPIC Dot Product
  dsPIC_SQRT : Subsystem  AncestorBlock=SLUGS_Library/dsPIC_SQRT
  Norm : Outport
  wires:
  dsPIC_SQRT/1(sqrt(x)) -> Norm/1
  Vector/1 -> dsPIC Dot Product/2, dsPIC Dot Product/1
  dsPIC Dot Product/1 -> dsPIC_SQRT/1(x)

== system AUAV_V3_TestSensors/Inner Loop/ Navigation/Navigation Encaps [updated 4.28.16]/Navigation/Normal WP  Navigation/On WP Enable/Subsystem/Compute Frenet/Normalize Vector ==
  Vector : Inport
  Divide : Product  Inputs=*/
  Vector Norm : Subsystem  AncestorBlock=SLUGS_Library/Vector Norm
  Zero Bound : Saturate  UpperLimit=inf  LowerLimit=0.001
  Normalized : Outport
  wires:
  Vector/1 -> Vector Norm/1(Vector), Divide/1
  Vector Norm/1(Norm) -> Zero Bound/1
  Zero Bound/1 -> Divide/2
  Divide/1 -> Normalized/1

== system AUAV_V3_TestSensors/Inner Loop/ Navigation/Navigation Encaps [updated 4.28.16]/Navigation/Normal WP  Navigation/On WP Enable/Subsystem/Compute Frenet/Normalize Vector  ==
  Vector : Inport
  Divide : Product  Inputs=*/
  Vector Norm : Subsystem  AncestorBlock=SLUGS_Library/Vector Norm
  Zero Bound : Saturate  UpperLimit=inf  LowerLimit=0.001
  Normalized : Outport
  wires:
  Vector/1 -> Vector Norm/1(Vector), Divide/1
  Vector Norm/1(Norm) -> Zero Bound/1
  Zero Bound/1 -> Divide/2
  Divide/1 -> Normalized/1

== system AUAV_V3_TestSensors/Inner Loop/ Navigation/Navigation Encaps [updated 4.28.16]/Navigation/Normal WP  Navigation/On WP Enable/Subsystem/get WP Coord from Index/Get WP from idx SIM ==
  GS LLA : Inport
  GS ECEF : Inport  Port=2
  idx : Inport  Port=3
  Constant : Constant  Value=latlong_WP  OutDataTypeStr=uint8  SampleTime=0.01
  Constant1 : Constant  Value=Ypoints  OutDataTypeStr=double  SampleTime=0.01
  Constant2 : Constant  Value=Xpoints  OutDataTypeStr=double  SampleTime=0.01
  Constant3 : Constant  Value=Zpoints  OutDataTypeStr=double  SampleTime=0.01
  Data Type Conversion : DataTypeConversion  OutDataTypeStr=double
  Data Type Conversion1 : DataTypeConversion  OutDataTypeStr=single
  Demux : Demux  Outputs=3
  Geod2LTP1 : SLUGS_Library/Navigation/Geod2LTP
  Mux : Mux  Inputs=3
  Switch : Switch  Criteria=u2 > Threshold  Threshold=0.3  ZeroCross=off
  Zero out Z1 : MATLAB Function  TreatAsAtomicUnit=on
  Zero out Z2 : MATLAB Function  TreatAsAtomicUnit=on
  Zero out Z3 : MATLAB Function  TreatAsAtomicUnit=on
  Out1 : Outport
  wires:
  Constant2/1 -> Zero out Z2/2(vect)
  Constant3/1 -> Zero out Z3/2(vect)
  Constant1/1 -> Zero out Z1/2(vect)
  Switch/1 -> Out1/1
  idx/1 -> Data Type Conversion/1
  GS ECEF/1 -> Geod2LTP1/2
  GS LLA/1 -> Geod2LTP1/1
  Data Type Conversion1/1 -> Demux/1, Switch/3
  Geod2LTP1/1 -> Switch/1
  Demux/3 -> Geod2LTP1/5
  Demux/2 -> Geod2LTP1/4
  Demux/1 -> Geod2LTP1/3
  Constant/1 -> Switch/2
  Mux/1 -> Data Type Conversion1/1
  Zero out Z3/1(y) -> Mux/3
  Zero out Z1/1(y) -> Mux/2
  Zero out Z2/1(y) -> Mux/1
  Data Type Conversion/1 -> Zero out Z3/1(idx), Zero out Z1/1(idx), Zero out Z2/1(idx)

== system AUAV_V3_TestSensors/Inner Loop/ Navigation/Navigation Encaps [updated 4.28.16]/Navigation/Normal WP  Navigation/On WP Enable/Subsystem/get WP Coord from Index1/Get WP from idx SIM ==
  GS LLA : Inport
  GS ECEF : Inport  Port=2
  idx : Inport  Port=3
  Constant : Constant  Value=latlong_WP  OutDataTypeStr=uint8  SampleTime=0.01
  Constant1 : Constant  Value=Ypoints  OutDataTypeStr=double  SampleTime=0.01
  Constant2 : Constant  Value=Xpoints  OutDataTypeStr=double  SampleTime=0.01
  Constant3 : Constant  Value=Zpoints  OutDataTypeStr=double  SampleTime=0.01
  Data Type Conversion : DataTypeConversion  OutDataTypeStr=double
  Data Type Conversion1 : DataTypeConversion  OutDataTypeStr=single
  Demux : Demux  Outputs=3
  Geod2LTP1 : SLUGS_Library/Navigation/Geod2LTP
  Mux : Mux  Inputs=3
  Switch : Switch  Criteria=u2 > Threshold  Threshold=0.3  ZeroCross=off
  Zero out Z1 : MATLAB Function  TreatAsAtomicUnit=on
  Zero out Z2 : MATLAB Function  TreatAsAtomicUnit=on
  Zero out Z3 : MATLAB Function  TreatAsAtomicUnit=on
  Out1 : Outport
  wires:
  Constant2/1 -> Zero out Z2/2(vect)
  Constant3/1 -> Zero out Z3/2(vect)
  Constant1/1 -> Zero out Z1/2(vect)
  Switch/1 -> Out1/1
  idx/1 -> Data Type Conversion/1
  GS ECEF/1 -> Geod2LTP1/2
  GS LLA/1 -> Geod2LTP1/1
  Data Type Conversion1/1 -> Demux/1, Switch/3
  Geod2LTP1/1 -> Switch/1
  Demux/3 -> Geod2LTP1/5
  Demux/2 -> Geod2LTP1/4
  Demux/1 -> Geod2LTP1/3
  Constant/1 -> Switch/2
  Mux/1 -> Data Type Conversion1/1
  Zero out Z3/1(y) -> Mux/3
  Zero out Z1/1(y) -> Mux/2
  Zero out Z2/1(y) -> Mux/1
  Data Type Conversion/1 -> Zero out Z3/1(idx), Zero out Z1/1(idx), Zero out Z2/1(idx)

== system AUAV_V3_TestSensors/Inner Loop/ Navigation/Navigation Encaps [updated 4.28.16]/Navigation/Recent Enable/Grab Upon Enable/Compute GS Location/Geod2ECEF1/eccentricity^2 ==
  " " : Product  OutDataTypeStr=single  SaturateOnIntegerOverflow=on  InputSameDT=on
  Re=equatorial radius1 : Constant  Value=Re  OutDataTypeStr=single
  Rp=polar radius : Constant  Value=Rp  OutDataTypeStr=single
  Sum5 : Sum  Inputs=|+-  SaturateOnIntegerOverflow=on  InputSameDT=on  OutDataTypeStr=Inherit: Same as first input
  const2 : Constant  OutDataTypeStr=single
  e^1 : Product  Inputs=*/  OutDataTypeStr=single  SaturateOnIntegerOverflow=on  InputSameDT=on
  e^2 : Outport
  wires:
  Re=equatorial radius1/1 -> e^1/2
  Rp=polar radius/1 -> e^1/1
  const2/1 -> Sum5/1
  e^1/1 -> " "/2, " "/1
  " "/1 -> Sum5/2
  Sum5/1 -> e^2/1

== system AUAV_V3_TestSensors/Inner Loop/ Navigation/Navigation Encaps [updated 4.28.16]/Navigation/Normal WP  Navigation/Get Frenet/Compute Frenet/Normalize Vector/Vector Norm/dsPIC_SQRT ==
  x : Inport
  Environment Controller : simulink/Signal Routing/Environment Controller
  Math Function1 : Math  Operator=sqrt  SaturateOnIntegerOverflow=on
  mySqrt() apUtils.c [updated 5.1.16] : MCHP_Blockset/User Functions/C Function Call  ParseFilesChkbx=off  ListFunctions1=Custom Function  Function1=float mySqrt(float x)  AddHeaderDeclaration=on  Function1Type=when block is updated (default)  Fct1BlockIn=x  FctReturnBlockOut=on  DataCollected=0  ORDERING=None  SampleTime=-1  MCHP_MASTERLINK=|  PinDigitalInput=[]  PinDigitalOutput=[]  PinAnalogInput=[]
      | AUAV_V3_TestSensors/Microchip Master
      | AUAV V3 Board
      | Busy Flag on D2 (RA6)
  negprotect : MATLAB Function  TreatAsAtomicUnit=on
  sqrt(x) : Outport
  wires:
  x/1 -> negprotect/1(val)
  negprotect/1(zpVal) -> Math Function1/1, mySqrt() apUtils.c [updated 5.1.16]/1
  Environment Controller/1 -> sqrt(x)/1
  Math Function1/1 -> Environment Controller/1
  mySqrt() apUtils.c [updated 5.1.16]/1 -> Environment Controller/2

== system AUAV_V3_TestSensors/Inner Loop/ Navigation/Navigation Encaps [updated 4.28.16]/Navigation/Normal WP  Navigation/Get Frenet/Compute Frenet/Normalize Vector /Vector Norm/dsPIC_SQRT ==
  x : Inport
  Environment Controller : simulink/Signal Routing/Environment Controller
  Math Function1 : Math  Operator=sqrt  SaturateOnIntegerOverflow=on
  mySqrt() apUtils.c [updated 5.1.16] : MCHP_Blockset/User Functions/C Function Call  ParseFilesChkbx=off  ListFunctions1=Custom Function  Function1=float mySqrt(float x)  AddHeaderDeclaration=on  Function1Type=when block is updated (default)  Fct1BlockIn=x  FctReturnBlockOut=on  DataCollected=0  ORDERING=None  SampleTime=-1  MCHP_MASTERLINK=|  PinDigitalInput=[]  PinDigitalOutput=[]  PinAnalogInput=[]
      | AUAV_V3_TestSensors/Microchip Master
      | AUAV V3 Board
      | Busy Flag on D2 (RA6)
  negprotect : MATLAB Function  TreatAsAtomicUnit=on
  sqrt(x) : Outport
  wires:
  x/1 -> negprotect/1(val)
  negprotect/1(zpVal) -> Math Function1/1, mySqrt() apUtils.c [updated 5.1.16]/1
  Environment Controller/1 -> sqrt(x)/1
  Math Function1/1 -> Environment Controller/1
  mySqrt() apUtils.c [updated 5.1.16]/1 -> Environment Controller/2

== system AUAV_V3_TestSensors/Inner Loop/ Navigation/Navigation Encaps [updated 4.28.16]/Navigation/Normal WP  Navigation/On WP Enable/Subsystem/Compute Frenet/Normalize Vector/Vector Norm ==
  Vector : Inport
  dsPIC Dot Product : SLUGS_Library/dsPIC Dot Product
  dsPIC_SQRT : Subsystem  AncestorBlock=SLUGS_Library/dsPIC_SQRT
  Norm : Outport
  wires:
  dsPIC_SQRT/1(sqrt(x)) -> Norm/1
  Vector/1 -> dsPIC Dot Product/2, dsPIC Dot Product/1
  dsPIC Dot Product/1 -> dsPIC_SQRT/1(x)

== system AUAV_V3_TestSensors/Inner Loop/ Navigation/Navigation Encaps [updated 4.28.16]/Navigation/Normal WP  Navigation/On WP Enable/Subsystem/Compute Frenet/Normalize Vector /Vector Norm ==
  Vector : Inport
  dsPIC Dot Product : SLUGS_Library/dsPIC Dot Product
  dsPIC_SQRT : Subsystem  AncestorBlock=SLUGS_Library/dsPIC_SQRT
  Norm : Outport
  wires:
  dsPIC_SQRT/1(sqrt(x)) -> Norm/1
  Vector/1 -> dsPIC Dot Product/2, dsPIC Dot Product/1
  dsPIC Dot Product/1 -> dsPIC_SQRT/1(x)

== system AUAV_V3_TestSensors/Inner Loop/ Navigation/Navigation Encaps [updated 4.28.16]/Navigation/Normal WP  Navigation/On WP Enable/Subsystem/Compute Frenet/Normalize Vector/Vector Norm/dsPIC_SQRT ==
  x : Inport
  Environment Controller : simulink/Signal Routing/Environment Controller
  Math Function1 : Math  Operator=sqrt  SaturateOnIntegerOverflow=on
  mySqrt() apUtils.c [updated 5.1.16] : MCHP_Blockset/User Functions/C Function Call  ParseFilesChkbx=off  ListFunctions1=Custom Function  Function1=float mySqrt(float x)  AddHeaderDeclaration=on  Function1Type=when block is updated (default)  Fct1BlockIn=x  FctReturnBlockOut=on  DataCollected=0  ORDERING=None  SampleTime=-1  MCHP_MASTERLINK=|  PinDigitalInput=[]  PinDigitalOutput=[]  PinAnalogInput=[]
      | AUAV_V3_TestSensors/Microchip Master
      | AUAV V3 Board
      | Busy Flag on D2 (RA6)
  negprotect : MATLAB Function  TreatAsAtomicUnit=on
  sqrt(x) : Outport
  wires:
  x/1 -> negprotect/1(val)
  negprotect/1(zpVal) -> Math Function1/1, mySqrt() apUtils.c [updated 5.1.16]/1
  Environment Controller/1 -> sqrt(x)/1
  Math Function1/1 -> Environment Controller/1
  mySqrt() apUtils.c [updated 5.1.16]/1 -> Environment Controller/2

== system AUAV_V3_TestSensors/Inner Loop/ Navigation/Navigation Encaps [updated 4.28.16]/Navigation/Normal WP  Navigation/On WP Enable/Subsystem/Compute Frenet/Normalize Vector /Vector Norm/dsPIC_SQRT ==
  x : Inport
  Environment Controller : simulink/Signal Routing/Environment Controller
  Math Function1 : Math  Operator=sqrt  SaturateOnIntegerOverflow=on
  mySqrt() apUtils.c [updated 5.1.16] : MCHP_Blockset/User Functions/C Function Call  ParseFilesChkbx=off  ListFunctions1=Custom Function  Function1=float mySqrt(float x)  AddHeaderDeclaration=on  Function1Type=when block is updated (default)  Fct1BlockIn=x  FctReturnBlockOut=on  DataCollected=0  ORDERING=None  SampleTime=-1  MCHP_MASTERLINK=|  PinDigitalInput=[]  PinDigitalOutput=[]  PinAnalogInput=[]
      | AUAV_V3_TestSensors/Microchip Master
      | AUAV V3 Board
      | Busy Flag on D2 (RA6)
  negprotect : MATLAB Function  TreatAsAtomicUnit=on
  sqrt(x) : Outport
  wires:
  x/1 -> negprotect/1(val)
  negprotect/1(zpVal) -> Math Function1/1, mySqrt() apUtils.c [updated 5.1.16]/1
  Environment Controller/1 -> sqrt(x)/1
  Math Function1/1 -> Environment Controller/1
  mySqrt() apUtils.c [updated 5.1.16]/1 -> Environment Controller/2

== matlab function Sensor_Data_Adapter/Sensor Suite/myMux Fun ==
  data: u1 input double; y output double; u2 input double; u3 input double
function y = myMux3(u1, u2, u3)
% This block supports an embeddable subset of the MATLAB language.
% See the help menu for details. 

y = [u1(1); u2(1); u3(1)];

== matlab function Position_and_Attitude_Filter/Position Filter/BlendPosVel/Subsystem/Embedded MATLAB Function1 ==
  data: u input double size=1; y output double size=1; NewGPS input double size=1; apSampleTime parameter double size=1
function y = RateAid(u,NewGPS,apSampleTime)
persistent LastU;
persistent TimeSinceLast;
persistent rate;
persistent OldRate;

if (isempty(LastU))
    LastU = single(0.);
    TimeSinceLast = single(apSampleTime);
    rate = single(0);
    OldRate = single(0);
end

if (NewGPS)
    OldRate = rate;
    rate = single((u - LastU)/TimeSinceLast);
    TimeSinceLast = single(0);
    LastU = u;
end
y = u + ( .5*rate + .5*OldRate )*TimeSinceLast;
TimeSinceLast = TimeSinceLast + apSampleTime;

== matlab function Position_and_Attitude_Filter/Position Filter/BlendPosVel/Subsystem/Embedded MATLAB Function2 ==
  data: u input double size=1; y output double size=1; NewGPS input double size=1; apSampleTime parameter double size=1
function y = RateAid(u,NewGPS,apSampleTime)
persistent LastU;
persistent TimeSinceLast;
persistent rate;
persistent OldRate;

if (isempty(LastU))
    LastU = single(0.);
    TimeSinceLast = single(apSampleTime);
    rate = single(0);
    OldRate = single(0);
end

if (NewGPS)
    OldRate = rate;
    rate = single((u - LastU)/TimeSinceLast);
    TimeSinceLast = single(0);
    LastU = u;
end
y = u + ( .5*rate + .5*OldRate )*TimeSinceLast;
TimeSinceLast = TimeSinceLast + apSampleTime;

== matlab function myMux Fun4 ==
  data: u1 input double; y output double; u2 input double
function y = myMux(u1, u2)
% This block supports an embeddable subset of the MATLAB language.
% See the help menu for details. 

y = [u1(1:3); u2(1:3)];

== matlab function myMux Fun3 ==
  data: u1 input double; y output double; u2 input double
function y = myMux(u1, u2)
% This block supports an embeddable subset of the MATLAB language.
% See the help menu for details. 

y = [u1(1:3); u2(1:3)];

== matlab function Position_and_Attitude_Filter/Position Filter/BlendPosVel/2 FIlter Blend/Embedded MATLAB Function3 ==
  data: gps_h input double size=1; h_rate output double size=1; NewGPS input double size=1; apSampleTime parameter double size=1; baseHeight input double
function h_rate = heightRateAid(gps_h,NewGPS,apSampleTime, baseHeight)
persistent lastGps_h;
persistent TimeSinceLast;
persistent rate;
% persistent lastH;

if (isempty(lastGps_h))
    lastGps_h       = single(0.0);
    TimeSinceLast   = single(apSampleTime);
    rate            = single(0);
%     lastH           = single(-baseHeight);
%     h_rate          = single(0);
end

if (NewGPS)
    rate = single((gps_h - lastGps_h)/TimeSinceLast);
    TimeSinceLast = single(0);
    if (rate > -10.6) && (rate < 17.67)
%         h = lastH + gps_h - lastGps_h;
        h_rate = rate;
    else
%         h = lastH;
        h_rate = single(0);
    end
    lastGps_h = gps_h;
else
%     h = lastH;
    h_rate = single(0);
end

TimeSinceLast = TimeSinceLast + apSampleTime;
% lastH = h;
%%%%%%%%%%%%%%%%%%%%%%%%%%%%%%%%%%%%%%%%%%%%%%%%%%%%%%%%%%%%5
% persistent lastGps_h;
% persistent TimeSinceLast;
% persistent rate;
% persistent lastH;
% 
% if (isempty(lastGps_h))
%     lastGps_h       = single(0.0);
%     TimeSinceLast   = single(apSampleTime);
%     rate            = single(0);
%     lastH           = single(-baseHeight);
%     h_rate          = single(0);
% end
% 
% if (NewGPS)
%     rate = single((gps_h - lastGps_h)/TimeSinceLast);
%     TimeSinceLast = single(0);
%     if (rate > -10.6) && (rate < 17.67)
%         h = lastH + gps_h - lastGps_h;
% %         h_rate = rate;
%     else
%         h = lastH;
% %         h_rate = single(0);
%     end
%     lastGps_h = gps_h;
% else
%     h = lastH;
% %     h_rate = single(0);
% end
% 
% TimeSinceLast = TimeSinceLast + apSampleTime;
% lastH = h;

== matlab function Position_and_Attitude_Filter/Attitude Complimentary Filter COG/3D Filter/myMux Fun1 ==
  data: u1 input double; y output double; u2 input double; u3 input double
function y = myMux(u1, u2, u3)
% This block supports an embeddable subset of the MATLAB language.
% See the help menu for details. 

y = [u1(1); u2(1); u3(1)];

== matlab function Sensor_Data_Adapter/Raw HIL Readings/MATLAB Function ==
  data: u input double; y output double
function y = changeVectorSize13(u)
%#codegen

y = u(1:13);

== matlab function Position_and_Attitude_Filter/Position Filter/BlendPosVel/2 FIlter Blend/Tustin Lowpass, Auto Initial Condition4/Embedded MATLAB Function ==
  data: u input double; y output double; T input double; f input double
function y = fcn(u,T,f)
% This block supports an embeddable subset of the MATLAB language.
% See the help menu for details. 

persistent a
persistent b
persistent y_km1
persistent u_km1
if isempty(a)
    %tf = [T*omega/(2+T*omega) T*omega/(2+T*omega)],[1 (T*omega-2)/(T*omega+2)]
    %tf = [a a],[1 -b]
    omega = 2*pi*f;
    a=T*omega/(2+T*omega);
    b=-(T*omega-2)/(T*omega+2);
    y_km1=u;
    u_km1=u;
end

y = a*(u+u_km1)+b*y_km1;
y_km1=y;
u_km1=u;

== matlab function Position_and_Attitude_Filter/Attitude Complimentary Filter COG/Normalize Vector1/Norm/Subsystem3/Embedded MATLAB Function ==
  data: x input double; y input double; xDoty output double
function xDoty = myDot(x,y)
% This block supports an embeddable subset of the MATLAB language.
% See the help menu for details. 

xDoty = x(1)*y(1) + x(2)*y(2) + x(3)*y(3);

== matlab function Position_and_Attitude_Filter/Attitude Complimentary Filter COG/Normalize Vector2/Norm/Subsystem2/negprotect ==
  data: val input double; zpVal output double
function zpVal = negProt(val)
% This block supports an embeddable subset of the MATLAB language.
% See the help menu for details. 

if val >= single(0.001)
    zpVal = val;
else
    zpVal = single(0.001);
end

== matlab function Position_and_Attitude_Filter/Attitude Complimentary Filter COG/Normalize Vector2/Norm/Subsystem3/Embedded MATLAB Function ==
  data: x input double; y input double; xDoty output double
function xDoty = myDot(x,y)
% This block supports an embeddable subset of the MATLAB language.
% See the help menu for details. 

xDoty = x(1)*y(1) + x(2)*y(2) + x(3)*y(3);

== matlab function myMux Fun5 ==
  data: u1 input double; y output double; u2 input double; u3 input double
function y = myMux(u1, u2, u3)
% This block supports an embeddable subset of the MATLAB language.
% See the help menu for details. 

y = [u1(1:3); u2(1:3); u3(1:3)];

== matlab function Sensor_Data_Adapter/Sensor Suite/ADIS16405 Signal Cond /3D Tustin Lowpass, Auto Initial Condition2/Embedded MATLAB Function ==
  data: u input double; y output double; T input double; f input double
function y = fcn(u,T,f)
% This block supports an embeddable subset of the MATLAB language.
% See the help menu for details. 

persistent a
persistent b
persistent y_km1
persistent u_km1
if isempty(a)
    %tf = [T*omega/(2+T*omega) T*omega/(2+T*omega)],[1 (T*omega-2)/(T*omega+2)]
    %tf = [a a],[1 -b]
    omega = 2*pi*f;
    a=T*omega/(2+T*omega);
    b=-(T*omega-2)/(T*omega+2);
    y_km1=u;
    u_km1=u;
end

y = a*(u+u_km1)+b*y_km1;
y_km1=y;
u_km1=u;

== matlab function myMux Fun2 ==
  data: u1 input double; y output double; u2 input double
function y = myMux(u1, u2)
% This block supports an embeddable subset of the MATLAB language.
% See the help menu for details. 

y = [u1(1:3); u2(1:3)];

== matlab function Position_and_Attitude_Filter/Attitude Complimentary Filter COG/q dot calc ==
  data: q input double size=4; om_hat input double; q_dot output single size=4
function q_dot = qXom(q,om_hat)
% This block supports an embeddable subset of the MATLAB language.
% See the help menu for details. 

	s = q(1,1);
    v = q(2:4,1);
    q_dot = single(zeros(4,1));
    q_dot(1,1) = -.5*v'*om_hat;
    q_dot(2:4,1) =  .5*[ s    -v(3) v(2); ...
                        v(3)  s    -v(1); ...
                       -v(2) v(1) s]*om_hat;

== matlab function Sensor_Data_Adapter/Sensor Suite/ADIS16405 Signal Cond /3D Tustin Lowpass, Auto Initial Condition2/Embedded MATLAB Function1 ==
  data: u input double; y output double; T input double; f input double
function y = fcn(u,T,f)
% This block supports an embeddable subset of the MATLAB language.
% See the help menu for details. 

persistent a
persistent b
persistent y_km1
persistent u_km1
if isempty(a)
    %tf = [T*omega/(2+T*omega) T*omega/(2+T*omega)],[1 (T*omega-2)/(T*omega+2)]
    %tf = [a a],[1 -b]
    omega = 2*pi*f;
    a=T*omega/(2+T*omega);
    b=-(T*omega-2)/(T*omega+2);
    y_km1=u;
    u_km1=u;
end

y = a*(u+u_km1)+b*y_km1;
y_km1=y;
u_km1=u;

== matlab function Position_and_Attitude_Filter/Position Filter/BlendPosVel/3D Filter/myMux Fun1 ==
  data: u1 input double; y output double; u2 input double; u3 input double
function y = myMux(u1, u2, u3)
% This block supports an embeddable subset of the MATLAB language.
% See the help menu for details. 

y = [u1(1); u2(1); u3(1)];

== matlab function Control Surface Input/PilotConsole/myMux Fun5 ==
  data: u1 input double; y output double; u2 input double; u3 input double; u4 input double; u5 input double
function y = myMux(u1, u2, u3, u4, u5)
% This block supports an embeddable subset of the MATLAB language.
% See the help menu for details. 

y = [u1(1); u2(1); u3(1); u4(1); u5(1)];
